simulink model "tirerotationaldynamics21"  (R2015b)
settings: Solver=FixedStepAuto  StartTime=0.0  StopTime=1  FixedStep=0.001  RelTol=1e-3
values from neighbouring files (symbols this model uses):
  C = [1 0]    [ssmodel.m]    (also in ssmodel2.m = [1 0 0])
  Ga = [E G]    [ssmodel2.m]
  P = dare(phi_aug, gamma_aug, Q, R)    [ecs.m]    (also in ssmodel2.m = [eval(p1sol) eval(p2sol) eval(p3sol); eval(p4sol) eval(p5sol)
  pol1 = 0.5    [ssmodel2.m]
  pol2 = 0.55    [ssmodel2.m]
undefined symbols (not defined in the file or in its folder): Ad2, Bd2, Cd2, Dd2
settings Model: Creator=ADMIN  LastModifiedBy=ADMIN

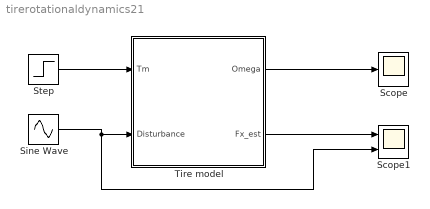
== system tirerotationaldynamics21 ==
  Scope : Scope
  Scope1 : Scope  NumInputPorts=2
  Sine Wave : Sin  Frequency=50
  Step : Step  Time=0.01
  Tire model : Subsystem  InitFcn=|
      | rw = 0.5;
      | Iw = 12.5;
      | pol1 = 0.5;
      | pol2 = 0.55;
      | A = [0 1 0; 0 0 -rw/Iw; 0 0 0];
      | B = [0 ; 1/Iw ; 0];
      | C = [1 0 0];
      | Do = 0;
      | Ts = 0.001;
      | 
      | systa = ss(A,B,C,Do);
      | systaa = c2d(systa, Ts);
      | Ad = systaa.a;
      | Bd = systaa.b;
      | Cd = systaa.c;
      | 
      | A2 = [ 0 1; 0 0 ];
      | B2 = [ 0 0; 1/Iw -rw/Iw];
      | C2 = [1 0];
      | D2 = [0 0];
      | 
      | sys2 = ss(A2,B2,C2,D2);
      | sysdis2 = c2d(sys2, Ts);
      | Ad2 = sysdis2.a;
      | Bd2 = sysdis2.b;
      | Cd2 = sysdis2.c;
      | Dd2 = sysdis2.d;
      | 
      | syms p1 p2 p3 p4 p5 p6; %unknowns
      | P = [p1 p2 p3; p4 p5 p6];
      | D = [0.5 0 ; 0 0.55];
      | G = [5 ; 10];%observer gain
      | [p1sol, p2sol, p3sol, p4sol, p5sol, p6sol] = solve(P*Ad - D*P == G*Cd);
      | P = [eval(p1sol) eval(p2sol) eval(p3sol); eval(p4sol) eval(p5sol) eval(p6sol)];
      | 
      | E = P*Bd;
      | 
      | Ga = [E G];
  wires:
  Sine Wave/1 -> Scope1/2, Tire model/2(Disturbance)
  Step/1 -> Tire model/1(Tm)
  Tire model/2(Fx_est) -> Scope1/1
  Tire model/1(Omega) -> Scope/1

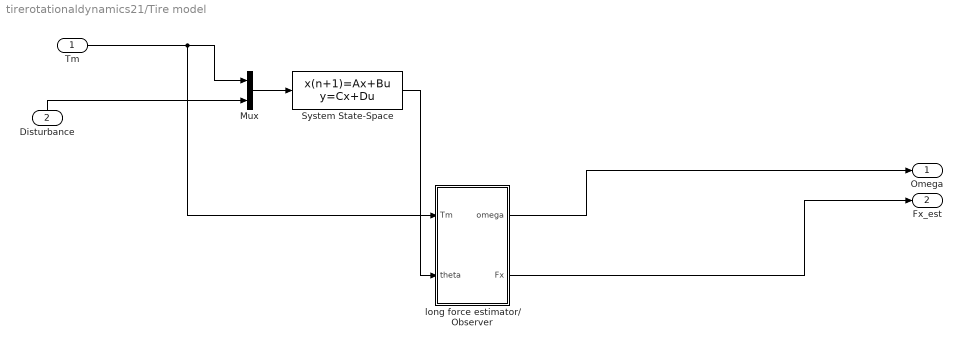
== system tirerotationaldynamics21/Tire model ==
  Tm : Inport
  Disturbance : Inport  Port=2
  Mux : Mux  Inputs=2
  System State-Space : DiscreteStateSpace  A=Ad2  B=Bd2  C=Cd2  D=Dd2  SampleTime=-1
  long force estimator/ Observer : Subsystem
  Omega : Outport
  Fx_est : Outport  Port=2
  wires:
  Tm/1 -> long force estimator/ Observer/1(Tm), Mux/1
  Mux/1 -> System State-Space/1
  Disturbance/1 -> Mux/2
  System State-Space/1 -> long force estimator/ Observer/2(theta)
  long force estimator/ Observer/1(omega) -> Omega/1
  long force estimator/ Observer/2(Fx) -> Fx_est/1

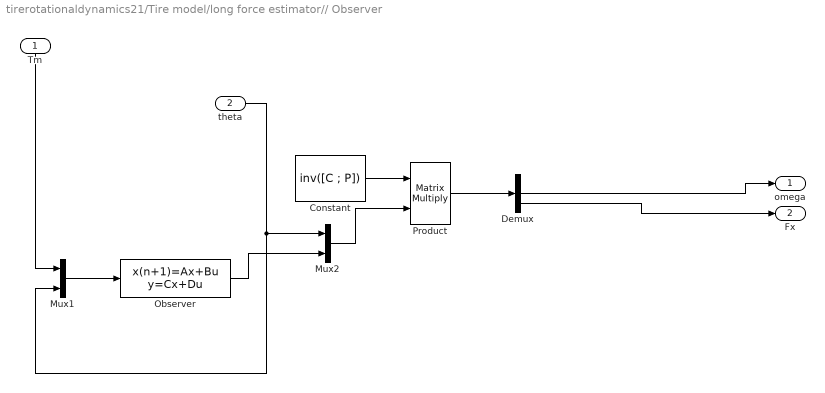
== system tirerotationaldynamics21/Tire model/long force estimator// Observer ==
  Tm : Inport
  theta : Inport  Port=2
  Constant : Constant  Value=inv([C ; P])
  Demux : Demux  Outputs=3
  Mux1 : Mux  Inputs=2
  Mux2 : Mux  Inputs=2
  Observer : DiscreteStateSpace  A=[pol1 0 ; 0 pol2]  B=Ga  C=[1 0; 0 1]  D=[0 0; 0 0]  SampleTime=-1
  Product : Product  Multiplication=Matrix(*)
  omega : Outport
  Fx : Outport  Port=2
  wires:
  Tm/1 -> Mux1/1
  Mux2/1 -> Product/2
  Demux/3 -> Fx/1
  Product/1 -> Demux/1
  Constant/1 -> Product/1
  theta/1 -> Mux2/1, Mux1/2
  Mux1/1 -> Observer/1
  Observer/1 -> Mux2/2
  Demux/2 -> omega/1
